simulink model "hybrid_control"  (R2016a)
settings: Solver=VariableStepAuto  StartTime=0.0  StopTime=1  RelTol=1e-4
undefined symbols (not defined in the file): K1, K2
settings Model: Creator=manuel  LastModifiedBy=manuel

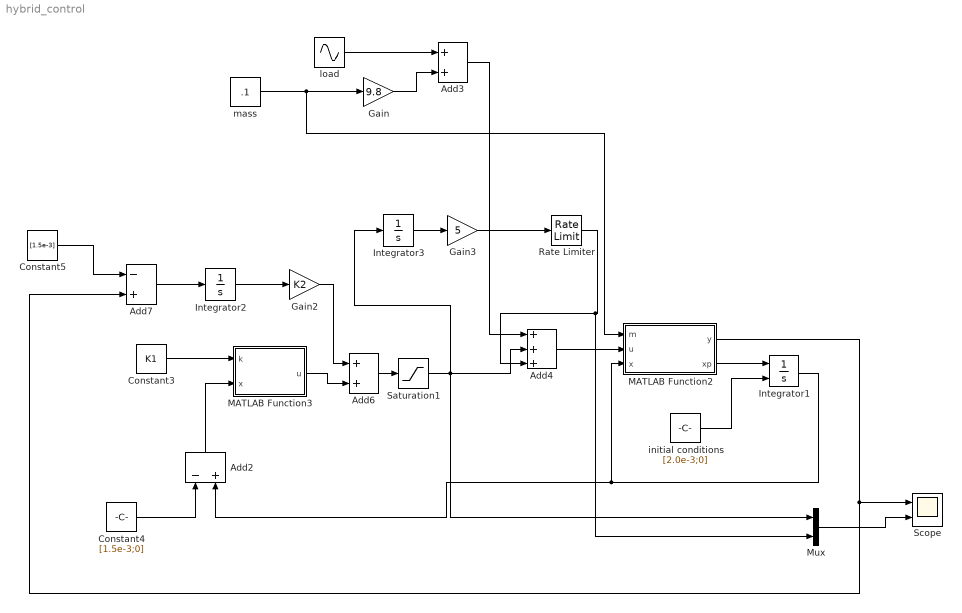
== system hybrid_control ==
  Add2 : Sum  Inputs=-+
  Add3 : Sum
  Add4 : Sum  Inputs=+++
  Add6 : Sum
  Add7 : Sum  Inputs=-+
  Constant3 : Constant  Value=K1
  Constant4 : Constant  Value=[1.5e-3;0]
  Constant5 : Constant  Value=[1.5e-3]
  Gain : Gain  Gain=9.8
  Gain2 : Gain  Gain=K2
  Gain3 : Gain  Gain=5
  Integrator1 : Integrator  InitialConditionSource=external  InitialCondition=[1.6e-3;0]  LimitOutput=on  UpperSaturationLimit=[2e-3;inf]  LowerSaturationLimit=[1e-3;-inf]
  Integrator2 : Integrator  InitialCondition=[0]  UpperSaturationLimit=[2e-3;inf]  LowerSaturationLimit=[1e-3;-inf]
  Integrator3 : Integrator  InitialCondition=[0]  UpperSaturationLimit=[2e-3;inf]  LowerSaturationLimit=[1e-3;-inf]
  MATLAB Function2 : MATLAB Function  TreatAsAtomicUnit=on
  MATLAB Function3 : MATLAB Function  TreatAsAtomicUnit=on
  Mux : Mux  Inputs=2
  Rate Limiter : RateLimiter  RisingSlewLimit=20  FallingSlewLimit=-20  SampleTimeMode=inherited
  Saturation1 : Saturate  UpperLimit=9.8  LowerLimit=-9.8
  Scope : Scope  NumInputPorts=2
  initial conditions : Constant  Value=[2.0e-3;0]
  load : Sin  Amplitude=2  Bias=4  Frequency=2*pi*100  SampleTime=0
  mass : Constant  Value=.1
  wires:
  Gain/1 -> Add3/2
  load/1 -> Add3/1
  MATLAB Function2/1(y) -> Scope/1, Add7/2
  MATLAB Function2/2(xp) -> Integrator1/1
  Integrator1/1 -> MATLAB Function2/3(x), Add2/2
  Constant3/1 -> MATLAB Function3/1(k)
  Constant4/1 -> Add2/1
  Add2/1 -> MATLAB Function3/2(x)
  Add4/1 -> MATLAB Function2/2(u)
  Add3/1 -> Add4/1
  initial conditions/1 -> Integrator1/2
  Integrator2/1 -> Gain2/1
  Add6/1 -> Saturation1/1
  Gain2/1 -> Add6/1
  MATLAB Function3/1(u) -> Add6/2
  Add7/1 -> Integrator2/1
  Constant5/1 -> Add7/1
  mass/1 -> Gain/1, MATLAB Function2/1(m)
  Integrator3/1 -> Gain3/1
  Gain3/1 -> Rate Limiter/1
  Rate Limiter/1 -> Mux/2, Add4/3
  Mux/1 -> Scope/2
  Saturation1/1 -> Mux/1, Integrator3/1, Add4/2

== matlab function hybrid_control/MATLAB Function2 ==
  data: m input; u input; x input; y output; xp output
function [y,xp] = mass_model(m,u,x)
%#codegen
A = [0 1
     0 0];
B = [0;
     1/m];
C = [1 0];

xp = A*x + B*u;
y = C*x;

== matlab function hybrid_control/MATLAB Function3 ==
  data: k input; x input; u output
function u = fcn(k,x)
%#codegen

u = -k'*x;
